simulink model "FuzzyTailv2"  (R2024b)
settings: Solver=VariableStepAuto  StartTime=0.0  StopTime=450  RelTol=1e-3
libraries: fuzblock x1
settings Model: Creator=ikostelidis  LastModifiedBy=ikostelidis

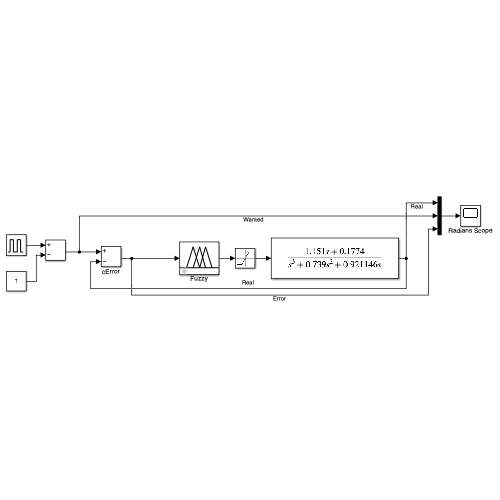
[thumbnail: Simulink's stored preview of the top-level diagram]
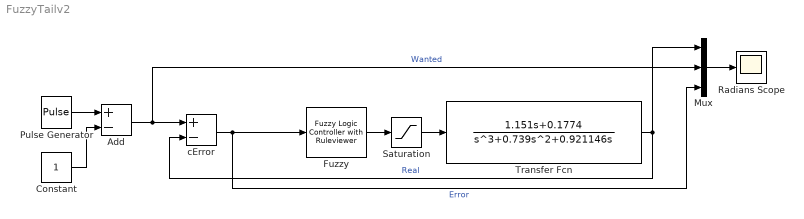
== system FuzzyTailv2 ==
  Add : Sum  Inputs=+-
  Constant : Constant
  Fuzzy : fuzblock/Fuzzy Logic  Controller  with Ruleviewer  fismatrix=FuzzyTailControl5v2  Ts=2
  Mux : Mux  Inputs=3
  Pulse Generator : DiscretePulseGenerator  PulseType=Time based  Amplitude=2  Period=500  PulseWidth=50
  Radians Scope : Scope
  Saturation : Saturate
  Transfer Fcn : TransferFcn  Numerator=[1.151 0.1774]  Denominator=[1 0.739 0.921146 0]
  cError : Sum  Inputs=+-
  wires:
  Saturation/1 -> Transfer Fcn/1
  Transfer Fcn/1 -> Mux/1, cError/2  "Real"
  Mux/1 -> Radians Scope/1
  Fuzzy/1 -> Saturation/1
  cError/1 -> Fuzzy/1, Mux/3  "Error"
  Add/1 -> cError/1, Mux/2  "Wanted"
  Pulse Generator/1 -> Add/1
  Constant/1 -> Add/2
